simulink model "fig3_connected"  (R2019b)
settings: Solver=VariableStepAuto  StartTime=0.0  StopTime=0.035  RelTol=1e-3
values from neighbouring files (symbols this model uses):
  C1 = 0    [Circuit_3_connected.m]    (also in Circuit_3_disconnected.m)
  C2 = 0    [Circuit_3_connected.m]    (also in Circuit_3_disconnected.m)
  C3 = 20e-6    (= 2e-05)    [Circuit_3_connected.m]    (also in Circuit_3_disconnected.m = 0)
  f = 50    [Circuit_1.m]    (also in Circuit_2.m; Circuit_3_connected.m; Circuit_3_disconnected.m)
  L1 = 1    [Circuit_3_connected.m]    (also in Circuit_3_disconnected.m)
  L2 = 0.5    [Circuit_3_connected.m]    (also in Circuit_3_disconnected.m = 1)
  L3 = 1    [Circuit_3_connected.m]    (also in Circuit_3_disconnected.m)
  R1 = 250    [Circuit_3_connected.m]    (also in Circuit_3_disconnected.m = 125)
  R2 = 125    [Circuit_3_connected.m]    (also in Circuit_3_disconnected.m = 62.5)
  R3 = 125    [Circuit_3_connected.m]    (also in Circuit_3_disconnected.m = 250)
  V = (400*sqrt(2))/sqrt(3)    [Circuit_1.m]    (also in Circuit_2.m; Circuit_3_connected.m = (70*sqrt(2))/sqrt(3); Circuit_3_disconnected.m = (70*sqrt(2))/sqrt(3))
libraries: powerlib x12
settings Model: Creator=100448597  LastModifiedBy=robom
settings DataIOCC: SaveOutput=off  ReturnWorkspaceOutputs=off
settings SFSimCC: CustomCodeUndefinedFunction=UseInterfaceOnly

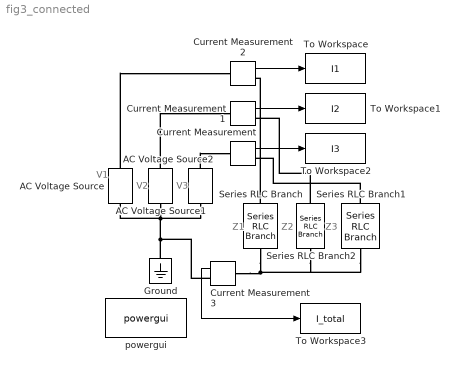
== system fig3_connected ==
  note: V1
  note: V2
  note: V3
  note: Z1
  note: Z2
  note: Z3
  AC Voltage Source : powerlib/Electrical Sources/AC Voltage Source  Amplitude=V  Phase=0  Frequency=f  SampleTime=0  Measurements=None  BusType=swing  Pref=10e3  Qref=0  Qmin=-inf  Qmax=+inf
      settings: SourceProductName=Simscape Electrical
  AC Voltage Source1 : powerlib/Electrical Sources/AC Voltage Source  Amplitude=V  Phase=-120  Frequency=f  SampleTime=0  Measurements=None  BusType=swing  Pref=10e3  Qref=0  Qmin=-inf  Qmax=+inf
      settings: SourceProductName=Simscape Electrical
  AC Voltage Source2 : powerlib/Electrical Sources/AC Voltage Source  Amplitude=V  Phase=-240  Frequency=f  SampleTime=0  Measurements=None  BusType=swing  Pref=10e3  Qref=0  Qmin=-inf  Qmax=+inf
      settings: SourceProductName=Simscape Electrical
  Current Measurement{,1..3} (4 alike) : powerlib/Measurements/Current Measurement  PhasorSimulation=off  OutputType=Complex  PSBequivalent=0
      settings: SourceProductName=Simscape Electrical
  Ground : powerlib/Elements/Ground  LConnTagsString=a
      settings: SourceProductName=Simscape Electrical
  Series RLC Branch : powerlib/Elements/Series RLC Branch  LConnTagsString=__new0  RConnTagsString=__new0  BranchType=RLC  Resistance=R1  Inductance=L1  SetiL0=on  InitialCurrent=0  Capacitance=C1  Setx0=off  InitialVoltage=0  Measurements=None
      settings: SourceProductName=Simscape Electrical
  Series RLC Branch1 : powerlib/Elements/Series RLC Branch  LConnTagsString=__new0  RConnTagsString=__new0  BranchType=RLC  Resistance=R3  Inductance=L3  SetiL0=on  InitialCurrent=0  Capacitance=C3  Setx0=off  InitialVoltage=0  Measurements=None
      settings: SourceProductName=Simscape Electrical
  Series RLC Branch2 : powerlib/Elements/Series RLC Branch  LConnTagsString=__new0  RConnTagsString=__new0  BranchType=RLC  Resistance=R2  Inductance=L2  SetiL0=on  InitialCurrent=0  Capacitance=C2  Setx0=off  InitialVoltage=0  Measurements=None
      settings: SourceProductName=Simscape Electrical
  To Workspace : ToWorkspace  VariableName=I1  SampleTime=-1
      settings: Save2DSignal=2-D array (concatenate along first dimension)
  To Workspace1 : ToWorkspace  VariableName=I2  SampleTime=-1
      settings: Save2DSignal=2-D array (concatenate along first dimension)
  To Workspace2 : ToWorkspace  VariableName=I3  SampleTime=-1
      settings: Save2DSignal=2-D array (concatenate along first dimension)
  To Workspace3 : ToWorkspace  VariableName=I_total  SampleTime=-1
      settings: Save2DSignal=2-D array (concatenate along first dimension)
  powergui : powerlib/powergui  Priority=1  SimulationMode=Continuous  SampleTime=50e-6  frequency=60  Iterations=50  frequencyindice=50  Pbase=100e6  ErrMax=1e-4  UnitsV=kV  UnitsW=MW  buscounter=0  FunctionMessages=off  echomessages=off  EnableUseOfTLC=off  CurrentSourceSwitches=off  DisableSnubberDevices=off  DisableRonSwitches=off  DisableVfSwitches=off  DisplayEquations=off  AutomaticDiscreteSolvers=off  SolverType=Tustin/Backward Euler (TBE)  Interpol=off  ExternalGateDelay=off  methode=off  Ts=100  x0status=blocks  SPID=on  SwTol=0  HookPort=off  NonlinearTolerance=0  nMaxIteration=15  ContinueOnMaxIteration=off  RestoreLinks=warning  ResistiveCurrentMeasurement=off  Frange=[0:2:500]  Ylog=off  Xlog=on  ShowGrid=off  save=off  variable=ZData  structure=0  ZoomFFT=off  StartTime=0.0  cycles=1  DisplayStyle=1  fundamental=60  FreqAxis=off  MaxFrequency=1000  frequencyindicesteady=1  RmsSteady=1  display=off
      settings: SourceProductName=Simscape Electrical
  wires:
  Current Measurement1/1 -> To Workspace1/1
  Current Measurement/1 -> To Workspace2/1
  Current Measurement2/1 -> To Workspace/1
  Current Measurement3/1 -> To Workspace3/1
  connections:
  Current Measurement3/LConn1 -- Series RLC Branch/RConn1 -- Series RLC Branch2/RConn1 -- Series RLC Branch1/RConn1
  Ground/LConn1 -- Current Measurement3/RConn1 -- AC Voltage Source2/LConn1 -- AC Voltage Source1/LConn1 -- AC Voltage Source/LConn1
  Series RLC Branch/LConn1 -- Current Measurement2/RConn1
  AC Voltage Source/RConn1 -- Current Measurement2/LConn1
  Series RLC Branch1/LConn1 -- Current Measurement/RConn1
  AC Voltage Source1/RConn1 -- Current Measurement1/LConn1
  AC Voltage Source2/RConn1 -- Current Measurement/LConn1
  Series RLC Branch2/LConn1 -- Current Measurement1/RConn1
